simulink model "TIE2019Simulation"  (R2016b)
settings: Solver=FixedStepAuto  StartTime=0.0  StopTime=100  FixedStep=0.01  RelTol=1e-3
InitFcn:
  | Disturbance_rotor_payload_ini;
StopFcn:
  | PlotResults;
values from neighbouring files (symbols this model uses):
  b1 = 220    [Disturbance_rotor_payload_ini.m]
  b2 = 110    [Disturbance_rotor_payload_ini.m]
  c_v = 1    [Disturbance_rotor_payload_ini.m]
  c_x = 1    [Disturbance_rotor_payload_ini.m]
  delta_W = 0*n    [Disturbance_rotor_payload_ini.m]
  g_I = [0 0 9.8]'    [Disturbance_rotor_payload_ini.m]
  invJ_B1 = inv(J)    [Disturbance_rotor_payload_ini.m]
  J = [2 0.3 -0.5;0.3 1 0.2;-0.5 0.2 3]*10^-2    [Disturbance_rotor_payload_ini.m]
  k = 0.6    [Disturbance_rotor_payload_ini.m]
  k_e = 15    [Disturbance_rotor_payload_ini.m]
  K_omega = 1*eye(3)    [Disturbance_rotor_payload_ini.m]
  K_q = 100    [Disturbance_rotor_payload_ini.m]
  K_R = 1*eye(3)    [Disturbance_rotor_payload_ini.m]
  k_v = 15    [Disturbance_rotor_payload_ini.m]
  L = 2    [Disturbance_rotor_payload_ini.m]
  Lambda_initalB01 = angle2quat(initial_Euler(3),initial_Euler(2),initial_Euler(1))    [Disturbance_rotor_payload_ini.m]
  lambda_p = 0.2    [Disturbance_rotor_payload_ini.m]
  lambda_q = 0.3    [Disturbance_rotor_payload_ini.m]
  lambda_theta = 1    [Disturbance_rotor_payload_ini.m]
  lambda_x = 1/20    (= 0.05)    [Disturbance_rotor_payload_ini.m]
  m_p = 2    [Disturbance_rotor_payload_ini.m]
  m_q = 2    [Disturbance_rotor_payload_ini.m]
  mid_point = (mid_point1+mid_point2)/2    [Disturbance_rotor_payload_ini.m]
  n = [n;0]    [Disturbance_rotor_payload_ini.m]
  n_ = n_/norm(n_)    [Disturbance_rotor_payload_ini.m]
  omega_b01 = [0.1 0.3 0]'    [Disturbance_rotor_payload_ini.m]
  sin_W = -5    [Disturbance_rotor_payload_ini.m]
  U_initial = [y_dot_initial;v_q]    [Disturbance_rotor_payload_ini.m]
  W_0 = (m_p+m_q)*v_q + m_p*B0*y_dot_initial    [Disturbance_rotor_payload_ini.m]
  W_p = [-3 3 -0.5]'    [Disturbance_rotor_payload_ini.m]
  W_q = [-5 4 -0.3]'    [Disturbance_rotor_payload_ini.m]
  waypoint_n = [n1 n2 n3 n4 n5]    [Disturbance_rotor_payload_ini.m]
  waypoint_p = [P1 P2 P3 P4 P5]    [Disturbance_rotor_payload_ini.m]
  waypoint_v = [v1 v2 v3 v4 v5]'    [Disturbance_rotor_payload_ini.m]
  X_initial = [0 0 0]'    [Disturbance_rotor_payload_ini.m]
  y_inital = [0.02 -0.02]'    [Disturbance_rotor_payload_ini.m]
libraries: aerolibtransform2 x4, dspmtrx3 x2, aerolibutil x2, dspinverses x2
(part 2 of 2)

== system TIE2019Simulation/Normal/Control_Force/Subsystem/Attitude Dynamics/Cross Matrix ==
  A : Inport
  Constant1 : Constant  Value=0  VectorParams1D=off
  Constant2 : Constant  Value=0  VectorParams1D=off
  Constant3 : Constant  Value=0  VectorParams1D=off
  Demux2 : Demux  Outputs=3
  Gain : Gain  Gain=-1
  Gain1 : Gain  Gain=-1
  Gain2 : Gain  Gain=-1
  Matrix Concatenate : Concatenate  NumInputs=3  Mode=Multidimensional array  ConcatenateDimension=2
  Matrix Concatenate1 : Concatenate  NumInputs=3  Mode=Multidimensional array
  Matrix Concatenate2 : Concatenate  NumInputs=3  Mode=Multidimensional array
  Matrix Concatenate3 : Concatenate  NumInputs=3  Mode=Multidimensional array
  AX : Outport
  wires:
  A/1 -> Demux2/1
  Demux2/1 -> Gain1/1, Matrix Concatenate2/3  "r1"
  Demux2/2 -> Gain2/1, Matrix Concatenate3/1  "r2"
  Matrix Concatenate/1 -> AX/1
  Demux2/3 -> Gain/1, Matrix Concatenate1/2  "r3"
  Matrix Concatenate1/1 -> Matrix Concatenate/1
  Matrix Concatenate2/1 -> Matrix Concatenate/2
  Constant2/1 -> Matrix Concatenate2/2
  Gain/1 -> Matrix Concatenate2/1
  Matrix Concatenate3/1 -> Matrix Concatenate/3
  Gain1/1 -> Matrix Concatenate3/2
  Constant3/1 -> Matrix Concatenate3/3
  Constant1/1 -> Matrix Concatenate1/1
  Gain2/1 -> Matrix Concatenate1/3

== system TIE2019Simulation/Normal/Control_Force/Subsystem/Attitude Dynamics/Quaternion Based Attitude Calculation ==
  OmegaBI,B : Inport
  Constant : Constant  Value=Lambda_initalB01
  Constant1 : Constant
  Dot Product : DotProduct  OutDataTypeStr=Inherit: Inherit via internal rule
  Gain : Gain  Gain=0.5
  Integrator : Integrator  InitialConditionSource=external
  L_hat : Subsystem
  Normalization Gain : Gain  Gain=K_q
  Product : Product  Multiplication=Matrix(*)  RndMeth=Zero
  Product1 : Product  RndMeth=Zero
  Quaternion Normalize : aerolibutil/Quaternion Normalize
  Quaternions to Direction Cosine Matrix : aerolibtransform2/Quaternions to  Direction Cosine Matrix
  Quaternions to Rotation Angles : aerolibtransform2/Quaternions to Rotation Angles  rotationOrder=ZYX
  Selector : Selector  InputPortWidth=3  IndexOptions=Index vector (dialog)  Indices=[3 2 1]  OutputSizes=1
  Sum : Sum  Inputs=|+-  SaturateOnIntegerOverflow=on  InputSameDT=on  OutDataTypeStr=Inherit: Same as first input
  Sum1 : Sum  Inputs=|++
  Transpose : Math  Operator=transpose  SaturateOnIntegerOverflow=on
  Transpose1 : Math  Operator=transpose  SaturateOnIntegerOverflow=on
  IRB : Outport
  BRI : Outport  Port=2
  Euler : Outport  Port=3
  wires:
  Constant/1 -> Integrator/2
  Quaternions to Rotation Angles/1 -> Selector/1
  Selector/1 -> Euler/1
  Integrator/1 -> Quaternion Normalize/1  "Lambda"
  Sum1/1 -> Integrator/1  "Lambda_dot"
  Quaternions to Direction Cosine Matrix/1 -> BRI/1, Transpose/1
  Transpose/1 -> IRB/1
  Dot Product/1 -> Sum/2
  Constant1/1 -> Sum/1
  L_hat/1(L_hat) -> Transpose1/1
  Transpose1/1 -> Product/1
  OmegaBI,B/1 -> Product/2
  Sum/1 -> Normalization Gain/1
  Product/1 -> Gain/1
  Gain/1 -> Sum1/1
  Normalization Gain/1 -> Product1/1
  Product1/1 -> Sum1/2
  Quaternion Normalize/1 -> Quaternions to Rotation Angles/1, Quaternions to Direction Cosine Matrix/1, Dot Product/1, Dot Product/2, L_hat/1(Lambda), Product1/2

== system TIE2019Simulation/Normal/Control_Force/Subsystem/Attitude Tracker/Cross Matrix ==
  A : Inport
  Constant1 : Constant  Value=0  VectorParams1D=off
  Constant2 : Constant  Value=0  VectorParams1D=off
  Constant3 : Constant  Value=0  VectorParams1D=off
  Demux2 : Demux  Outputs=3
  Gain : Gain  Gain=-1
  Gain1 : Gain  Gain=-1
  Gain2 : Gain  Gain=-1
  Matrix Concatenate : Concatenate  NumInputs=3  Mode=Multidimensional array  ConcatenateDimension=2
  Matrix Concatenate1 : Concatenate  NumInputs=3  Mode=Multidimensional array
  Matrix Concatenate2 : Concatenate  NumInputs=3  Mode=Multidimensional array
  Matrix Concatenate3 : Concatenate  NumInputs=3  Mode=Multidimensional array
  AX : Outport
  wires:
  A/1 -> Demux2/1
  Demux2/1 -> Gain1/1, Matrix Concatenate2/3  "r1"
  Demux2/2 -> Gain2/1, Matrix Concatenate3/1  "r2"
  Matrix Concatenate/1 -> AX/1
  Demux2/3 -> Gain/1, Matrix Concatenate1/2  "r3"
  Matrix Concatenate1/1 -> Matrix Concatenate/1
  Matrix Concatenate2/1 -> Matrix Concatenate/2
  Constant2/1 -> Matrix Concatenate2/2
  Gain/1 -> Matrix Concatenate2/1
  Matrix Concatenate3/1 -> Matrix Concatenate/3
  Gain1/1 -> Matrix Concatenate3/2
  Constant3/1 -> Matrix Concatenate3/3
  Constant1/1 -> Matrix Concatenate1/1
  Gain2/1 -> Matrix Concatenate1/3

== system TIE2019Simulation/Normal/Control_Force/Subsystem/Attitude Tracker/Cross Matrix1 ==
  A : Inport
  Constant1 : Constant  Value=0  VectorParams1D=off
  Constant2 : Constant  Value=0  VectorParams1D=off
  Constant3 : Constant  Value=0  VectorParams1D=off
  Demux2 : Demux  Outputs=3
  Gain : Gain  Gain=-1
  Gain1 : Gain  Gain=-1
  Gain2 : Gain  Gain=-1
  Matrix Concatenate : Concatenate  NumInputs=3  Mode=Multidimensional array  ConcatenateDimension=2
  Matrix Concatenate1 : Concatenate  NumInputs=3  Mode=Multidimensional array
  Matrix Concatenate2 : Concatenate  NumInputs=3  Mode=Multidimensional array
  Matrix Concatenate3 : Concatenate  NumInputs=3  Mode=Multidimensional array
  AX : Outport
  wires:
  A/1 -> Demux2/1
  Demux2/1 -> Gain1/1, Matrix Concatenate2/3  "r1"
  Demux2/2 -> Gain2/1, Matrix Concatenate3/1  "r2"
  Matrix Concatenate/1 -> AX/1
  Demux2/3 -> Gain/1, Matrix Concatenate1/2  "r3"
  Matrix Concatenate1/1 -> Matrix Concatenate/1
  Matrix Concatenate2/1 -> Matrix Concatenate/2
  Constant2/1 -> Matrix Concatenate2/2
  Gain/1 -> Matrix Concatenate2/1
  Matrix Concatenate3/1 -> Matrix Concatenate/3
  Gain1/1 -> Matrix Concatenate3/2
  Constant3/1 -> Matrix Concatenate3/3
  Constant1/1 -> Matrix Concatenate1/1
  Gain2/1 -> Matrix Concatenate1/3

== system TIE2019Simulation/Normal/Control_Force/Subsystem/Attitude Tracker/Cross Matrix2 ==
  A : Inport
  Constant1 : Constant  Value=0  VectorParams1D=off
  Constant2 : Constant  Value=0  VectorParams1D=off
  Constant3 : Constant  Value=0  VectorParams1D=off
  Demux2 : Demux  Outputs=3
  Gain : Gain  Gain=-1
  Gain1 : Gain  Gain=-1
  Gain2 : Gain  Gain=-1
  Matrix Concatenate : Concatenate  NumInputs=3  Mode=Multidimensional array  ConcatenateDimension=2
  Matrix Concatenate1 : Concatenate  NumInputs=3  Mode=Multidimensional array
  Matrix Concatenate2 : Concatenate  NumInputs=3  Mode=Multidimensional array
  Matrix Concatenate3 : Concatenate  NumInputs=3  Mode=Multidimensional array
  AX : Outport
  wires:
  A/1 -> Demux2/1
  Demux2/1 -> Gain1/1, Matrix Concatenate2/3  "r1"
  Demux2/2 -> Gain2/1, Matrix Concatenate3/1  "r2"
  Matrix Concatenate/1 -> AX/1
  Demux2/3 -> Gain/1, Matrix Concatenate1/2  "r3"
  Matrix Concatenate1/1 -> Matrix Concatenate/1
  Matrix Concatenate2/1 -> Matrix Concatenate/2
  Constant2/1 -> Matrix Concatenate2/2
  Gain/1 -> Matrix Concatenate2/1
  Matrix Concatenate3/1 -> Matrix Concatenate/3
  Gain1/1 -> Matrix Concatenate3/2
  Constant3/1 -> Matrix Concatenate3/3
  Constant1/1 -> Matrix Concatenate1/1
  Gain2/1 -> Matrix Concatenate1/3

== system TIE2019Simulation/Normal/Control_Force/Subsystem/Attitude Tracker/Cross Matrix3 ==
  A : Inport
  Constant1 : Constant  Value=0  VectorParams1D=off
  Constant2 : Constant  Value=0  VectorParams1D=off
  Constant3 : Constant  Value=0  VectorParams1D=off
  Demux2 : Demux  Outputs=3
  Gain : Gain  Gain=-1
  Gain1 : Gain  Gain=-1
  Gain2 : Gain  Gain=-1
  Matrix Concatenate : Concatenate  NumInputs=3  Mode=Multidimensional array  ConcatenateDimension=2
  Matrix Concatenate1 : Concatenate  NumInputs=3  Mode=Multidimensional array
  Matrix Concatenate2 : Concatenate  NumInputs=3  Mode=Multidimensional array
  Matrix Concatenate3 : Concatenate  NumInputs=3  Mode=Multidimensional array
  AX : Outport
  wires:
  A/1 -> Demux2/1
  Demux2/1 -> Gain1/1, Matrix Concatenate2/3  "r1"
  Demux2/2 -> Gain2/1, Matrix Concatenate3/1  "r2"
  Matrix Concatenate/1 -> AX/1
  Demux2/3 -> Gain/1, Matrix Concatenate1/2  "r3"
  Matrix Concatenate1/1 -> Matrix Concatenate/1
  Matrix Concatenate2/1 -> Matrix Concatenate/2
  Constant2/1 -> Matrix Concatenate2/2
  Gain/1 -> Matrix Concatenate2/1
  Matrix Concatenate3/1 -> Matrix Concatenate/3
  Gain1/1 -> Matrix Concatenate3/2
  Constant3/1 -> Matrix Concatenate3/3
  Constant1/1 -> Matrix Concatenate1/1
  Gain2/1 -> Matrix Concatenate1/3

== system TIE2019Simulation/Normal/Control_Force/Subsystem/Attitude Tracker/Cross Matrix4 ==
  A : Inport
  Constant1 : Constant  Value=0  VectorParams1D=off
  Constant2 : Constant  Value=0  VectorParams1D=off
  Constant3 : Constant  Value=0  VectorParams1D=off
  Demux2 : Demux  Outputs=3
  Gain : Gain  Gain=-1
  Gain1 : Gain  Gain=-1
  Gain2 : Gain  Gain=-1
  Matrix Concatenate : Concatenate  NumInputs=3  Mode=Multidimensional array  ConcatenateDimension=2
  Matrix Concatenate1 : Concatenate  NumInputs=3  Mode=Multidimensional array
  Matrix Concatenate2 : Concatenate  NumInputs=3  Mode=Multidimensional array
  Matrix Concatenate3 : Concatenate  NumInputs=3  Mode=Multidimensional array
  AX : Outport
  wires:
  A/1 -> Demux2/1
  Demux2/1 -> Gain1/1, Matrix Concatenate2/3  "r1"
  Demux2/2 -> Gain2/1, Matrix Concatenate3/1  "r2"
  Matrix Concatenate/1 -> AX/1
  Demux2/3 -> Gain/1, Matrix Concatenate1/2  "r3"
  Matrix Concatenate1/1 -> Matrix Concatenate/1
  Matrix Concatenate2/1 -> Matrix Concatenate/2
  Constant2/1 -> Matrix Concatenate2/2
  Gain/1 -> Matrix Concatenate2/1
  Matrix Concatenate3/1 -> Matrix Concatenate/3
  Gain1/1 -> Matrix Concatenate3/2
  Constant3/1 -> Matrix Concatenate3/3
  Constant1/1 -> Matrix Concatenate1/1
  Gain2/1 -> Matrix Concatenate1/3

== system TIE2019Simulation/Normal/Control_Force/Subsystem/Attitude Tracker/Cross Matrix5 ==
  A : Inport
  Constant1 : Constant  Value=0  VectorParams1D=off
  Constant2 : Constant  Value=0  VectorParams1D=off
  Constant3 : Constant  Value=0  VectorParams1D=off
  Demux2 : Demux  Outputs=3
  Gain : Gain  Gain=-1
  Gain1 : Gain  Gain=-1
  Gain2 : Gain  Gain=-1
  Matrix Concatenate : Concatenate  NumInputs=3  Mode=Multidimensional array  ConcatenateDimension=2
  Matrix Concatenate1 : Concatenate  NumInputs=3  Mode=Multidimensional array
  Matrix Concatenate2 : Concatenate  NumInputs=3  Mode=Multidimensional array
  Matrix Concatenate3 : Concatenate  NumInputs=3  Mode=Multidimensional array
  AX : Outport
  wires:
  A/1 -> Demux2/1
  Demux2/1 -> Gain1/1, Matrix Concatenate2/3  "r1"
  Demux2/2 -> Gain2/1, Matrix Concatenate3/1  "r2"
  Matrix Concatenate/1 -> AX/1
  Demux2/3 -> Gain/1, Matrix Concatenate1/2  "r3"
  Matrix Concatenate1/1 -> Matrix Concatenate/1
  Matrix Concatenate2/1 -> Matrix Concatenate/2
  Constant2/1 -> Matrix Concatenate2/2
  Gain/1 -> Matrix Concatenate2/1
  Matrix Concatenate3/1 -> Matrix Concatenate/3
  Gain1/1 -> Matrix Concatenate3/2
  Constant3/1 -> Matrix Concatenate3/3
  Constant1/1 -> Matrix Concatenate1/1
  Gain2/1 -> Matrix Concatenate1/3

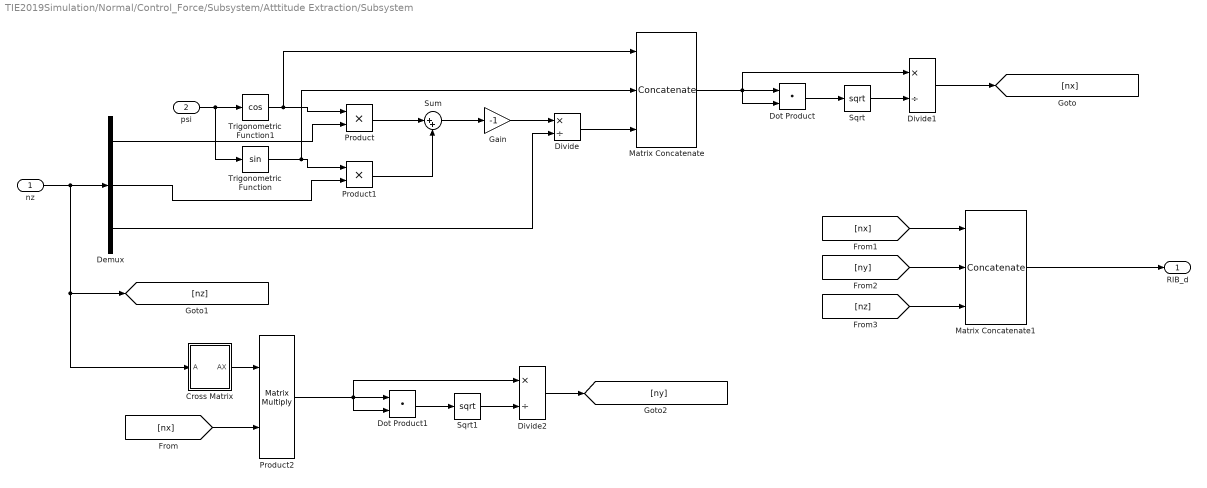
== system TIE2019Simulation/Normal/Control_Force/Subsystem/Atttitude Extraction/Subsystem ==
  nz : Inport
  psi : Inport  Port=2
  Cross Matrix : Subsystem
  Demux : Demux  Outputs=3
  Divide : Product  Inputs=*/
  Divide1 : Product  Inputs=*/
  Divide2 : Product  Inputs=*/
  Dot Product : DotProduct  InputSameDT=on  OutDataTypeStr=Inherit: Inherit via internal rule
  Dot Product1 : DotProduct  InputSameDT=on  OutDataTypeStr=Inherit: Inherit via internal rule
  Gain : Gain  Gain=-1
  Matrix Concatenate : Concatenate  NumInputs=3  Mode=Multidimensional array
  Matrix Concatenate1 : Concatenate  NumInputs=3  Mode=Multidimensional array  ConcatenateDimension=2
  Product : Product
  Product1 : Product
  Product2 : Product  Multiplication=Matrix(*)
  Sqrt : Sqrt  SaturateOnIntegerOverflow=on
  Sqrt1 : Sqrt  SaturateOnIntegerOverflow=on
  Sum : Sum  Inputs=|++
  Trigonometric Function : Trigonometry
  Trigonometric Function1 : Trigonometry  Operator=cos
  RIB_d : Outport
  wires:
  nz/1 -> Cross Matrix/1(A), [nz], Demux/1
  Demux/1 -> Product/2
  Demux/3 -> Divide/2
  psi/1 -> Trigonometric Function/1, Trigonometric Function1/1
  Trigonometric Function1/1 -> Matrix Concatenate/1, Product/1
  Trigonometric Function/1 -> Matrix Concatenate/2, Product1/1
  Demux/2 -> Product1/2
  Product/1 -> Sum/1
  Product1/1 -> Sum/2
  Sum/1 -> Gain/1
  Gain/1 -> Divide/1
  Divide/1 -> Matrix Concatenate/3
  Matrix Concatenate/1 -> Divide1/1, Dot Product/1, Dot Product/2
  Dot Product/1 -> Sqrt/1
  Sqrt/1 -> Divide1/2
  Divide1/1 -> [nx]
  Cross Matrix/1(AX) -> Product2/1
  [nx] -> Product2/2
  [nx] -> Matrix Concatenate1/1
  [ny] -> Matrix Concatenate1/2
  [nz] -> Matrix Concatenate1/3
  Product2/1 -> Divide2/1, Dot Product1/1, Dot Product1/2
  Dot Product1/1 -> Sqrt1/1
  Sqrt1/1 -> Divide2/2
  Divide2/1 -> [ny]
  Matrix Concatenate1/1 -> RIB_d/1

== system TIE2019Simulation/Normal/Control_Force/Subsystem/Atttitude Extraction/vee map ==
  skrew symmetric matrix : Inport
  Display2 : Display
  Display3 : Display
  Mux : Mux  Inputs=3
  Selector : Selector  NumberOfDimensions=2  InputPortWidth=3  IndexOptions=Index vector (dialog),Index vector (dialog)  Indices=3,2  OutputSizes=1,1
  Selector1 : Selector  NumberOfDimensions=2  InputPortWidth=3  IndexOptions=Index vector (dialog),Index vector (dialog)  Indices=1,3  OutputSizes=1,1
  Selector2 : Selector  NumberOfDimensions=2  InputPortWidth=3  IndexOptions=Index vector (dialog),Index vector (dialog)  Indices=2,1  OutputSizes=1,1
  phi : Outport
  wires:
  skrew symmetric matrix/1 -> Selector/1, Display3/1, Selector2/1, Selector1/1
  Mux/1 -> phi/1, Display2/1
  Selector/1 -> Mux/1
  Selector1/1 -> Mux/2
  Selector2/1 -> Mux/3

== system TIE2019Simulation/UDE/Control_Force/Subsystem/Attitude Dynamics/Cross Matrix ==
  A : Inport
  Constant1 : Constant  Value=0  VectorParams1D=off
  Constant2 : Constant  Value=0  VectorParams1D=off
  Constant3 : Constant  Value=0  VectorParams1D=off
  Demux2 : Demux  Outputs=3
  Gain : Gain  Gain=-1
  Gain1 : Gain  Gain=-1
  Gain2 : Gain  Gain=-1
  Matrix Concatenate : Concatenate  NumInputs=3  Mode=Multidimensional array  ConcatenateDimension=2
  Matrix Concatenate1 : Concatenate  NumInputs=3  Mode=Multidimensional array
  Matrix Concatenate2 : Concatenate  NumInputs=3  Mode=Multidimensional array
  Matrix Concatenate3 : Concatenate  NumInputs=3  Mode=Multidimensional array
  AX : Outport
  wires:
  A/1 -> Demux2/1
  Demux2/1 -> Gain1/1, Matrix Concatenate2/3  "r1"
  Demux2/2 -> Gain2/1, Matrix Concatenate3/1  "r2"
  Matrix Concatenate/1 -> AX/1
  Demux2/3 -> Gain/1, Matrix Concatenate1/2  "r3"
  Matrix Concatenate1/1 -> Matrix Concatenate/1
  Matrix Concatenate2/1 -> Matrix Concatenate/2
  Constant2/1 -> Matrix Concatenate2/2
  Gain/1 -> Matrix Concatenate2/1
  Matrix Concatenate3/1 -> Matrix Concatenate/3
  Gain1/1 -> Matrix Concatenate3/2
  Constant3/1 -> Matrix Concatenate3/3
  Constant1/1 -> Matrix Concatenate1/1
  Gain2/1 -> Matrix Concatenate1/3

== system TIE2019Simulation/UDE/Control_Force/Subsystem/Attitude Dynamics/Quaternion Based Attitude Calculation ==
  OmegaBI,B : Inport
  Constant : Constant  Value=Lambda_initalB01
  Constant1 : Constant
  Dot Product : DotProduct  OutDataTypeStr=Inherit: Inherit via internal rule
  Gain : Gain  Gain=0.5
  Integrator : Integrator  InitialConditionSource=external
  L_hat : Subsystem
  Normalization Gain : Gain  Gain=K_q
  Product : Product  Multiplication=Matrix(*)  RndMeth=Zero
  Product1 : Product  RndMeth=Zero
  Quaternion Normalize : aerolibutil/Quaternion Normalize
  Quaternions to Direction Cosine Matrix : aerolibtransform2/Quaternions to  Direction Cosine Matrix
  Quaternions to Rotation Angles : aerolibtransform2/Quaternions to Rotation Angles  rotationOrder=ZYX
  Selector : Selector  InputPortWidth=3  IndexOptions=Index vector (dialog)  Indices=[3 2 1]  OutputSizes=1
  Sum : Sum  Inputs=|+-  SaturateOnIntegerOverflow=on  InputSameDT=on  OutDataTypeStr=Inherit: Same as first input
  Sum1 : Sum  Inputs=|++
  Transpose : Math  Operator=transpose  SaturateOnIntegerOverflow=on
  Transpose1 : Math  Operator=transpose  SaturateOnIntegerOverflow=on
  IRB : Outport
  BRI : Outport  Port=2
  Euler : Outport  Port=3
  wires:
  Constant/1 -> Integrator/2
  Quaternions to Rotation Angles/1 -> Selector/1
  Selector/1 -> Euler/1
  Integrator/1 -> Quaternion Normalize/1  "Lambda"
  Sum1/1 -> Integrator/1  "Lambda_dot"
  Quaternions to Direction Cosine Matrix/1 -> BRI/1, Transpose/1
  Transpose/1 -> IRB/1
  Dot Product/1 -> Sum/2
  Constant1/1 -> Sum/1
  L_hat/1(L_hat) -> Transpose1/1
  Transpose1/1 -> Product/1
  OmegaBI,B/1 -> Product/2
  Sum/1 -> Normalization Gain/1
  Product/1 -> Gain/1
  Gain/1 -> Sum1/1
  Normalization Gain/1 -> Product1/1
  Product1/1 -> Sum1/2
  Quaternion Normalize/1 -> Quaternions to Rotation Angles/1, Quaternions to Direction Cosine Matrix/1, Dot Product/1, Dot Product/2, L_hat/1(Lambda), Product1/2

== system TIE2019Simulation/UDE/Control_Force/Subsystem/Attitude Tracker/Cross Matrix ==
  A : Inport
  Constant1 : Constant  Value=0  VectorParams1D=off
  Constant2 : Constant  Value=0  VectorParams1D=off
  Constant3 : Constant  Value=0  VectorParams1D=off
  Demux2 : Demux  Outputs=3
  Gain : Gain  Gain=-1
  Gain1 : Gain  Gain=-1
  Gain2 : Gain  Gain=-1
  Matrix Concatenate : Concatenate  NumInputs=3  Mode=Multidimensional array  ConcatenateDimension=2
  Matrix Concatenate1 : Concatenate  NumInputs=3  Mode=Multidimensional array
  Matrix Concatenate2 : Concatenate  NumInputs=3  Mode=Multidimensional array
  Matrix Concatenate3 : Concatenate  NumInputs=3  Mode=Multidimensional array
  AX : Outport
  wires:
  A/1 -> Demux2/1
  Demux2/1 -> Gain1/1, Matrix Concatenate2/3  "r1"
  Demux2/2 -> Gain2/1, Matrix Concatenate3/1  "r2"
  Matrix Concatenate/1 -> AX/1
  Demux2/3 -> Gain/1, Matrix Concatenate1/2  "r3"
  Matrix Concatenate1/1 -> Matrix Concatenate/1
  Matrix Concatenate2/1 -> Matrix Concatenate/2
  Constant2/1 -> Matrix Concatenate2/2
  Gain/1 -> Matrix Concatenate2/1
  Matrix Concatenate3/1 -> Matrix Concatenate/3
  Gain1/1 -> Matrix Concatenate3/2
  Constant3/1 -> Matrix Concatenate3/3
  Constant1/1 -> Matrix Concatenate1/1
  Gain2/1 -> Matrix Concatenate1/3

== system TIE2019Simulation/UDE/Control_Force/Subsystem/Attitude Tracker/Cross Matrix1 ==
  A : Inport
  Constant1 : Constant  Value=0  VectorParams1D=off
  Constant2 : Constant  Value=0  VectorParams1D=off
  Constant3 : Constant  Value=0  VectorParams1D=off
  Demux2 : Demux  Outputs=3
  Gain : Gain  Gain=-1
  Gain1 : Gain  Gain=-1
  Gain2 : Gain  Gain=-1
  Matrix Concatenate : Concatenate  NumInputs=3  Mode=Multidimensional array  ConcatenateDimension=2
  Matrix Concatenate1 : Concatenate  NumInputs=3  Mode=Multidimensional array
  Matrix Concatenate2 : Concatenate  NumInputs=3  Mode=Multidimensional array
  Matrix Concatenate3 : Concatenate  NumInputs=3  Mode=Multidimensional array
  AX : Outport
  wires:
  A/1 -> Demux2/1
  Demux2/1 -> Gain1/1, Matrix Concatenate2/3  "r1"
  Demux2/2 -> Gain2/1, Matrix Concatenate3/1  "r2"
  Matrix Concatenate/1 -> AX/1
  Demux2/3 -> Gain/1, Matrix Concatenate1/2  "r3"
  Matrix Concatenate1/1 -> Matrix Concatenate/1
  Matrix Concatenate2/1 -> Matrix Concatenate/2
  Constant2/1 -> Matrix Concatenate2/2
  Gain/1 -> Matrix Concatenate2/1
  Matrix Concatenate3/1 -> Matrix Concatenate/3
  Gain1/1 -> Matrix Concatenate3/2
  Constant3/1 -> Matrix Concatenate3/3
  Constant1/1 -> Matrix Concatenate1/1
  Gain2/1 -> Matrix Concatenate1/3

== system TIE2019Simulation/UDE/Control_Force/Subsystem/Attitude Tracker/Cross Matrix2 ==
  A : Inport
  Constant1 : Constant  Value=0  VectorParams1D=off
  Constant2 : Constant  Value=0  VectorParams1D=off
  Constant3 : Constant  Value=0  VectorParams1D=off
  Demux2 : Demux  Outputs=3
  Gain : Gain  Gain=-1
  Gain1 : Gain  Gain=-1
  Gain2 : Gain  Gain=-1
  Matrix Concatenate : Concatenate  NumInputs=3  Mode=Multidimensional array  ConcatenateDimension=2
  Matrix Concatenate1 : Concatenate  NumInputs=3  Mode=Multidimensional array
  Matrix Concatenate2 : Concatenate  NumInputs=3  Mode=Multidimensional array
  Matrix Concatenate3 : Concatenate  NumInputs=3  Mode=Multidimensional array
  AX : Outport
  wires:
  A/1 -> Demux2/1
  Demux2/1 -> Gain1/1, Matrix Concatenate2/3  "r1"
  Demux2/2 -> Gain2/1, Matrix Concatenate3/1  "r2"
  Matrix Concatenate/1 -> AX/1
  Demux2/3 -> Gain/1, Matrix Concatenate1/2  "r3"
  Matrix Concatenate1/1 -> Matrix Concatenate/1
  Matrix Concatenate2/1 -> Matrix Concatenate/2
  Constant2/1 -> Matrix Concatenate2/2
  Gain/1 -> Matrix Concatenate2/1
  Matrix Concatenate3/1 -> Matrix Concatenate/3
  Gain1/1 -> Matrix Concatenate3/2
  Constant3/1 -> Matrix Concatenate3/3
  Constant1/1 -> Matrix Concatenate1/1
  Gain2/1 -> Matrix Concatenate1/3

== system TIE2019Simulation/UDE/Control_Force/Subsystem/Attitude Tracker/Cross Matrix3 ==
  A : Inport
  Constant1 : Constant  Value=0  VectorParams1D=off
  Constant2 : Constant  Value=0  VectorParams1D=off
  Constant3 : Constant  Value=0  VectorParams1D=off
  Demux2 : Demux  Outputs=3
  Gain : Gain  Gain=-1
  Gain1 : Gain  Gain=-1
  Gain2 : Gain  Gain=-1
  Matrix Concatenate : Concatenate  NumInputs=3  Mode=Multidimensional array  ConcatenateDimension=2
  Matrix Concatenate1 : Concatenate  NumInputs=3  Mode=Multidimensional array
  Matrix Concatenate2 : Concatenate  NumInputs=3  Mode=Multidimensional array
  Matrix Concatenate3 : Concatenate  NumInputs=3  Mode=Multidimensional array
  AX : Outport
  wires:
  A/1 -> Demux2/1
  Demux2/1 -> Gain1/1, Matrix Concatenate2/3  "r1"
  Demux2/2 -> Gain2/1, Matrix Concatenate3/1  "r2"
  Matrix Concatenate/1 -> AX/1
  Demux2/3 -> Gain/1, Matrix Concatenate1/2  "r3"
  Matrix Concatenate1/1 -> Matrix Concatenate/1
  Matrix Concatenate2/1 -> Matrix Concatenate/2
  Constant2/1 -> Matrix Concatenate2/2
  Gain/1 -> Matrix Concatenate2/1
  Matrix Concatenate3/1 -> Matrix Concatenate/3
  Gain1/1 -> Matrix Concatenate3/2
  Constant3/1 -> Matrix Concatenate3/3
  Constant1/1 -> Matrix Concatenate1/1
  Gain2/1 -> Matrix Concatenate1/3

== system TIE2019Simulation/UDE/Control_Force/Subsystem/Attitude Tracker/Cross Matrix4 ==
  A : Inport
  Constant1 : Constant  Value=0  VectorParams1D=off
  Constant2 : Constant  Value=0  VectorParams1D=off
  Constant3 : Constant  Value=0  VectorParams1D=off
  Demux2 : Demux  Outputs=3
  Gain : Gain  Gain=-1
  Gain1 : Gain  Gain=-1
  Gain2 : Gain  Gain=-1
  Matrix Concatenate : Concatenate  NumInputs=3  Mode=Multidimensional array  ConcatenateDimension=2
  Matrix Concatenate1 : Concatenate  NumInputs=3  Mode=Multidimensional array
  Matrix Concatenate2 : Concatenate  NumInputs=3  Mode=Multidimensional array
  Matrix Concatenate3 : Concatenate  NumInputs=3  Mode=Multidimensional array
  AX : Outport
  wires:
  A/1 -> Demux2/1
  Demux2/1 -> Gain1/1, Matrix Concatenate2/3  "r1"
  Demux2/2 -> Gain2/1, Matrix Concatenate3/1  "r2"
  Matrix Concatenate/1 -> AX/1
  Demux2/3 -> Gain/1, Matrix Concatenate1/2  "r3"
  Matrix Concatenate1/1 -> Matrix Concatenate/1
  Matrix Concatenate2/1 -> Matrix Concatenate/2
  Constant2/1 -> Matrix Concatenate2/2
  Gain/1 -> Matrix Concatenate2/1
  Matrix Concatenate3/1 -> Matrix Concatenate/3
  Gain1/1 -> Matrix Concatenate3/2
  Constant3/1 -> Matrix Concatenate3/3
  Constant1/1 -> Matrix Concatenate1/1
  Gain2/1 -> Matrix Concatenate1/3

== system TIE2019Simulation/UDE/Control_Force/Subsystem/Attitude Tracker/Cross Matrix5 ==
  A : Inport
  Constant1 : Constant  Value=0  VectorParams1D=off
  Constant2 : Constant  Value=0  VectorParams1D=off
  Constant3 : Constant  Value=0  VectorParams1D=off
  Demux2 : Demux  Outputs=3
  Gain : Gain  Gain=-1
  Gain1 : Gain  Gain=-1
  Gain2 : Gain  Gain=-1
  Matrix Concatenate : Concatenate  NumInputs=3  Mode=Multidimensional array  ConcatenateDimension=2
  Matrix Concatenate1 : Concatenate  NumInputs=3  Mode=Multidimensional array
  Matrix Concatenate2 : Concatenate  NumInputs=3  Mode=Multidimensional array
  Matrix Concatenate3 : Concatenate  NumInputs=3  Mode=Multidimensional array
  AX : Outport
  wires:
  A/1 -> Demux2/1
  Demux2/1 -> Gain1/1, Matrix Concatenate2/3  "r1"
  Demux2/2 -> Gain2/1, Matrix Concatenate3/1  "r2"
  Matrix Concatenate/1 -> AX/1
  Demux2/3 -> Gain/1, Matrix Concatenate1/2  "r3"
  Matrix Concatenate1/1 -> Matrix Concatenate/1
  Matrix Concatenate2/1 -> Matrix Concatenate/2
  Constant2/1 -> Matrix Concatenate2/2
  Gain/1 -> Matrix Concatenate2/1
  Matrix Concatenate3/1 -> Matrix Concatenate/3
  Gain1/1 -> Matrix Concatenate3/2
  Constant3/1 -> Matrix Concatenate3/3
  Constant1/1 -> Matrix Concatenate1/1
  Gain2/1 -> Matrix Concatenate1/3

== system TIE2019Simulation/UDE/Control_Force/Subsystem/Atttitude Extraction/Subsystem ==
  nz : Inport
  psi : Inport  Port=2
  Cross Matrix : Subsystem
  Demux : Demux  Outputs=3
  Divide : Product  Inputs=*/
  Divide1 : Product  Inputs=*/
  Divide2 : Product  Inputs=*/
  Dot Product : DotProduct  InputSameDT=on  OutDataTypeStr=Inherit: Inherit via internal rule
  Dot Product1 : DotProduct  InputSameDT=on  OutDataTypeStr=Inherit: Inherit via internal rule
  Gain : Gain  Gain=-1
  Matrix Concatenate : Concatenate  NumInputs=3  Mode=Multidimensional array
  Matrix Concatenate1 : Concatenate  NumInputs=3  Mode=Multidimensional array  ConcatenateDimension=2
  Product : Product
  Product1 : Product
  Product2 : Product  Multiplication=Matrix(*)
  Sqrt : Sqrt  SaturateOnIntegerOverflow=on
  Sqrt1 : Sqrt  SaturateOnIntegerOverflow=on
  Sum : Sum  Inputs=|++
  Trigonometric Function : Trigonometry
  Trigonometric Function1 : Trigonometry  Operator=cos
  RIB_d : Outport
  wires:
  nz/1 -> Cross Matrix/1(A), [nz], Demux/1
  Demux/1 -> Product/2
  Demux/3 -> Divide/2
  psi/1 -> Trigonometric Function/1, Trigonometric Function1/1
  Trigonometric Function1/1 -> Matrix Concatenate/1, Product/1
  Trigonometric Function/1 -> Matrix Concatenate/2, Product1/1
  Demux/2 -> Product1/2
  Product/1 -> Sum/1
  Product1/1 -> Sum/2
  Sum/1 -> Gain/1
  Gain/1 -> Divide/1
  Divide/1 -> Matrix Concatenate/3
  Matrix Concatenate/1 -> Divide1/1, Dot Product/1, Dot Product/2
  Dot Product/1 -> Sqrt/1
  Sqrt/1 -> Divide1/2
  Divide1/1 -> [nx]
  Cross Matrix/1(AX) -> Product2/1
  [nx] -> Product2/2
  [nx] -> Matrix Concatenate1/1
  [ny] -> Matrix Concatenate1/2
  [nz] -> Matrix Concatenate1/3
  Product2/1 -> Divide2/1, Dot Product1/1, Dot Product1/2
  Dot Product1/1 -> Sqrt1/1
  Sqrt1/1 -> Divide2/2
  Divide2/1 -> [ny]
  Matrix Concatenate1/1 -> RIB_d/1

== system TIE2019Simulation/UDE/Control_Force/Subsystem/Atttitude Extraction/vee map ==
  skrew symmetric matrix : Inport
  Display2 : Display
  Display3 : Display
  Mux : Mux  Inputs=3
  Selector : Selector  NumberOfDimensions=2  InputPortWidth=3  IndexOptions=Index vector (dialog),Index vector (dialog)  Indices=3,2  OutputSizes=1,1
  Selector1 : Selector  NumberOfDimensions=2  InputPortWidth=3  IndexOptions=Index vector (dialog),Index vector (dialog)  Indices=1,3  OutputSizes=1,1
  Selector2 : Selector  NumberOfDimensions=2  InputPortWidth=3  IndexOptions=Index vector (dialog),Index vector (dialog)  Indices=2,1  OutputSizes=1,1
  phi : Outport
  wires:
  skrew symmetric matrix/1 -> Selector/1, Display3/1, Selector2/1, Selector1/1
  Mux/1 -> phi/1, Display2/1
  Selector/1 -> Mux/1
  Selector1/1 -> Mux/2
  Selector2/1 -> Mux/3

== system TIE2019Simulation/Normal/Control_Force/Subsystem/Attitude Dynamics/Quaternion Based Attitude Calculation/L_hat ==
  Lambda : Inport
  Create Diagonal Matrix : dspmtrx3/Create Diagonal Matrix
  Cross Matrix : Subsystem
  Gain : Gain  Gain=-1
  Gain1 : Gain  Gain=[1 1 1]
  Gain2 : Gain  Gain=-1
  Matrix Concatenate : Concatenate  Mode=Multidimensional array  ConcatenateDimension=2
  Selector : Selector  InputPortWidth=4  IndexOptions=Index vector (dialog)  Indices=[2 3 4]  OutputSizes=1
  Selector1 : Selector  InputPortWidth=4  IndexOptions=Index vector (dialog)  Indices=[1]  OutputSizes=1
  Sum : Sum  Inputs=|++
  L_hat : Outport
  wires:
  Lambda/1 -> Selector/1, Selector1/1
  Gain/1 -> Matrix Concatenate/1
  Matrix Concatenate/1 -> L_hat/1
  Cross Matrix/1(AX) -> Gain2/1  "LambdaX"
  Sum/1 -> Matrix Concatenate/2
  Selector1/1 -> Gain1/1
  Gain1/1 -> Create Diagonal Matrix/1
  Selector/1 -> Cross Matrix/1(A), Gain/1
  Create Diagonal Matrix/1 -> Sum/2
  Gain2/1 -> Sum/1

== system TIE2019Simulation/Normal/Control_Force/Subsystem/Atttitude Extraction/Subsystem/Cross Matrix ==
  A : Inport
  Constant1 : Constant  Value=0  VectorParams1D=off
  Constant2 : Constant  Value=0  VectorParams1D=off
  Constant3 : Constant  Value=0  VectorParams1D=off
  Demux2 : Demux  Outputs=3
  Gain : Gain  Gain=-1
  Gain1 : Gain  Gain=-1
  Gain2 : Gain  Gain=-1
  Matrix Concatenate : Concatenate  NumInputs=3  Mode=Multidimensional array  ConcatenateDimension=2
  Matrix Concatenate1 : Concatenate  NumInputs=3  Mode=Multidimensional array
  Matrix Concatenate2 : Concatenate  NumInputs=3  Mode=Multidimensional array
  Matrix Concatenate3 : Concatenate  NumInputs=3  Mode=Multidimensional array
  AX : Outport
  wires:
  A/1 -> Demux2/1
  Demux2/1 -> Gain1/1, Matrix Concatenate2/3  "r1"
  Demux2/2 -> Gain2/1, Matrix Concatenate3/1  "r2"
  Matrix Concatenate/1 -> AX/1
  Demux2/3 -> Gain/1, Matrix Concatenate1/2  "r3"
  Matrix Concatenate1/1 -> Matrix Concatenate/1
  Matrix Concatenate2/1 -> Matrix Concatenate/2
  Constant2/1 -> Matrix Concatenate2/2
  Gain/1 -> Matrix Concatenate2/1
  Matrix Concatenate3/1 -> Matrix Concatenate/3
  Gain1/1 -> Matrix Concatenate3/2
  Constant3/1 -> Matrix Concatenate3/3
  Constant1/1 -> Matrix Concatenate1/1
  Gain2/1 -> Matrix Concatenate1/3

== system TIE2019Simulation/UDE/Control_Force/Subsystem/Attitude Dynamics/Quaternion Based Attitude Calculation/L_hat ==
  Lambda : Inport
  Create Diagonal Matrix : dspmtrx3/Create Diagonal Matrix
  Cross Matrix : Subsystem
  Gain : Gain  Gain=-1
  Gain1 : Gain  Gain=[1 1 1]
  Gain2 : Gain  Gain=-1
  Matrix Concatenate : Concatenate  Mode=Multidimensional array  ConcatenateDimension=2
  Selector : Selector  InputPortWidth=4  IndexOptions=Index vector (dialog)  Indices=[2 3 4]  OutputSizes=1
  Selector1 : Selector  InputPortWidth=4  IndexOptions=Index vector (dialog)  Indices=[1]  OutputSizes=1
  Sum : Sum  Inputs=|++
  L_hat : Outport
  wires:
  Lambda/1 -> Selector/1, Selector1/1
  Gain/1 -> Matrix Concatenate/1
  Matrix Concatenate/1 -> L_hat/1
  Cross Matrix/1(AX) -> Gain2/1  "LambdaX"
  Sum/1 -> Matrix Concatenate/2
  Selector1/1 -> Gain1/1
  Gain1/1 -> Create Diagonal Matrix/1
  Selector/1 -> Cross Matrix/1(A), Gain/1
  Create Diagonal Matrix/1 -> Sum/2
  Gain2/1 -> Sum/1

== system TIE2019Simulation/UDE/Control_Force/Subsystem/Atttitude Extraction/Subsystem/Cross Matrix ==
  A : Inport
  Constant1 : Constant  Value=0  VectorParams1D=off
  Constant2 : Constant  Value=0  VectorParams1D=off
  Constant3 : Constant  Value=0  VectorParams1D=off
  Demux2 : Demux  Outputs=3
  Gain : Gain  Gain=-1
  Gain1 : Gain  Gain=-1
  Gain2 : Gain  Gain=-1
  Matrix Concatenate : Concatenate  NumInputs=3  Mode=Multidimensional array  ConcatenateDimension=2
  Matrix Concatenate1 : Concatenate  NumInputs=3  Mode=Multidimensional array
  Matrix Concatenate2 : Concatenate  NumInputs=3  Mode=Multidimensional array
  Matrix Concatenate3 : Concatenate  NumInputs=3  Mode=Multidimensional array
  AX : Outport
  wires:
  A/1 -> Demux2/1
  Demux2/1 -> Gain1/1, Matrix Concatenate2/3  "r1"
  Demux2/2 -> Gain2/1, Matrix Concatenate3/1  "r2"
  Matrix Concatenate/1 -> AX/1
  Demux2/3 -> Gain/1, Matrix Concatenate1/2  "r3"
  Matrix Concatenate1/1 -> Matrix Concatenate/1
  Matrix Concatenate2/1 -> Matrix Concatenate/2
  Constant2/1 -> Matrix Concatenate2/2
  Gain/1 -> Matrix Concatenate2/1
  Matrix Concatenate3/1 -> Matrix Concatenate/3
  Gain1/1 -> Matrix Concatenate3/2
  Constant3/1 -> Matrix Concatenate3/3
  Constant1/1 -> Matrix Concatenate1/1
  Gain2/1 -> Matrix Concatenate1/3

== system TIE2019Simulation/Normal/Control_Force/Subsystem/Attitude Dynamics/Quaternion Based Attitude Calculation/L_hat/Cross Matrix ==
  A : Inport
  Constant1 : Constant  Value=0
  Constant2 : Constant  Value=0
  Constant3 : Constant  Value=0
  Demux2 : Demux  Outputs=3
  Gain : Gain  Gain=-1
  Gain1 : Gain  Gain=-1
  Gain2 : Gain  Gain=-1
  Matrix Concatenate : Concatenate  NumInputs=3  Mode=Multidimensional array  ConcatenateDimension=2
  Mux : Mux  Inputs=3
  Mux1 : Mux  Inputs=3
  Mux2 : Mux  Inputs=3
  AX : Outport
  wires:
  A/1 -> Demux2/1
  Demux2/1 -> Mux1/3, Gain1/1  "r1"
  Demux2/2 -> Mux2/1, Gain2/1  "r2"
  Matrix Concatenate/1 -> AX/1
  Demux2/3 -> Gain/1, Mux/2  "r3"
  Mux/1 -> Matrix Concatenate/1
  Mux1/1 -> Matrix Concatenate/2
  Constant2/1 -> Mux1/2
  Gain/1 -> Mux1/1
  Mux2/1 -> Matrix Concatenate/3
  Gain1/1 -> Mux2/2
  Constant3/1 -> Mux2/3
  Constant1/1 -> Mux/1
  Gain2/1 -> Mux/3

== system TIE2019Simulation/UDE/Control_Force/Subsystem/Attitude Dynamics/Quaternion Based Attitude Calculation/L_hat/Cross Matrix ==
  A : Inport
  Constant1 : Constant  Value=0
  Constant2 : Constant  Value=0
  Constant3 : Constant  Value=0
  Demux2 : Demux  Outputs=3
  Gain : Gain  Gain=-1
  Gain1 : Gain  Gain=-1
  Gain2 : Gain  Gain=-1
  Matrix Concatenate : Concatenate  NumInputs=3  Mode=Multidimensional array  ConcatenateDimension=2
  Mux : Mux  Inputs=3
  Mux1 : Mux  Inputs=3
  Mux2 : Mux  Inputs=3
  AX : Outport
  wires:
  A/1 -> Demux2/1
  Demux2/1 -> Mux1/3, Gain1/1  "r1"
  Demux2/2 -> Mux2/1, Gain2/1  "r2"
  Matrix Concatenate/1 -> AX/1
  Demux2/3 -> Gain/1, Mux/2  "r3"
  Mux/1 -> Matrix Concatenate/1
  Mux1/1 -> Matrix Concatenate/2
  Constant2/1 -> Mux1/2
  Gain/1 -> Mux1/1
  Mux2/1 -> Matrix Concatenate/3
  Gain1/1 -> Mux2/2
  Constant3/1 -> Mux2/3
  Constant1/1 -> Mux/1
  Gain2/1 -> Mux/3

== stateflow chart TIE2019Simulation/Normal/Control_Force/Chart ==
  state Initialization
    entry:
    index = initial_value;
    WayPoint_ni = reshape(WayPoint_n(:,index),3,1);
    WayPoint_Pi = reshape(WayPoint_P(:,index),3,1);
    WayPoint_vi =  WayPoint_v(index);
    flag=0;
    NUM_waypoints = max(size(WayPoint_v));
    position_error1 = 0;
  state Error
    during:
    if index<NUM_waypoints
    position_error1 = norm(Position-reshape(WayPoint_P(:,index+1),3,1));
    if position_error1<= WayPoint_v(index)*3
    flag=1;
    end
    else
    flag=0;
    end
  state INSIDE
    entry:
    index = index +1;
    WayPoint_ni = reshape(WayPoint_n(:,index),3,1);
    WayPoint_Pi = reshape(WayPoint_P(:,index),3,1);
    WayPoint_vi =  WayPoint_v(index);
    flag=0;
  (default) -> Initialization
  Initialization -> Error
  Error -> INSIDE : [flag==1]
  INSIDE -> Error : [flag==0]
  data: Position input; initial_value input; WayPoint_Pi output; WayPoint_ni output; WayPoint_P input; WayPoint_n input; index local; WayPoint_v input; WayPoint_vi output; flag local double size=1; position_error1 local; NUM_waypoints local

== stateflow chart TIE2019Simulation/UDE/Control_Force/Chart ==
  state Initialization
    entry:
    index = initial_value;
    WayPoint_ni = reshape(WayPoint_n(:,index),3,1);
    WayPoint_Pi = reshape(WayPoint_P(:,index),3,1);
    WayPoint_vi =  WayPoint_v(index);
    flag=0;
    NUM_waypoints = max(size(WayPoint_v));
    position_error1 = 0;
  state Error
    during:
    if index<NUM_waypoints
    position_error1 = norm(Position-reshape(WayPoint_P(:,index+1),3,1));
    if position_error1<= WayPoint_v(index)*3
    flag=1;
    end
    else
    flag=0;
    end
  state INSIDE
    entry:
    index = index +1;
    WayPoint_ni = reshape(WayPoint_n(:,index),3,1);
    WayPoint_Pi = reshape(WayPoint_P(:,index),3,1);
    WayPoint_vi =  WayPoint_v(index);
    flag=0;
  (default) -> Initialization
  Initialization -> Error
  Error -> INSIDE : [flag==1]
  INSIDE -> Error : [flag==0]
  data: Position input; initial_value input; WayPoint_Pi output; WayPoint_ni output; WayPoint_P input; WayPoint_n input; index local; WayPoint_v input; WayPoint_vi output; flag local double size=1; position_error1 local; NUM_waypoints local
